simulink library "libEularAngleCalculator"  (R2016b)
settings: Solver=VariableStepAuto  StartTime=0.0  StopTime=10.0  RelTol=1e-3
libraries: simulink_extras x2
settings Model: Creator=vibek  LastModifiedBy=vibek

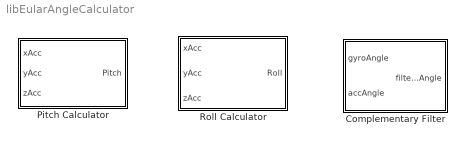
== system libEularAngleCalculator ==
  "Complementary Filter " : Subsystem
      mask DialogControl DescTextVar Prompt: Input Values of accelerometer and gyroscope angles to calculate filtered output angle
  Pitch Calculator : Subsystem  Description=takes 3 inputs from accelerometer and outputs pitch value
      settings: PermitHierarchicalResolution=None
      mask DialogControl DescTextVar Prompt: Input values of x, y, and z of Accelerometer data to calculate the value of Pitch
      mask Display: image('C:\Users\vibek\Pictures\93277-MG945-Servo-Motor-Metal-Gear-Tower-Pro-1-1200x630w.JPG');
  Roll Calculator : Subsystem  Description=takes 3 inputs from accelerometer and outputs pitch value
      mask DialogControl DescTextVar Prompt: Input values of x, y, and z of Accelerometer data to calculate the value of roll
      mask Display: image('C:\Users\vibek\Pictures\motor-tire.jpg');

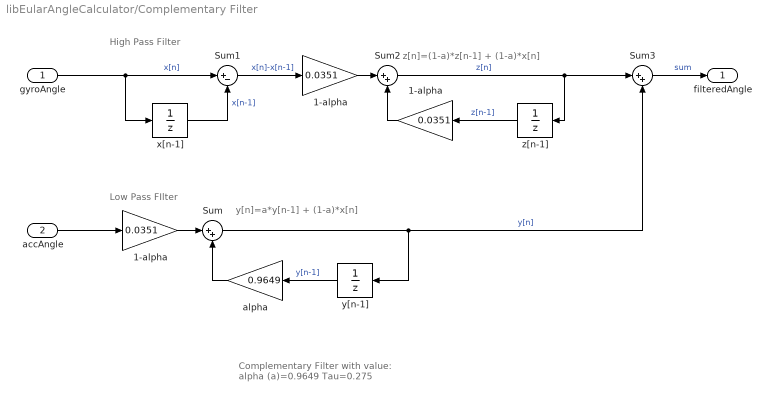
== system libEularAngleCalculator/Complementary Filter  ==
  note: Complementary Filter with value:
      | alpha (a)=0.9649
      | Tau=0.275
  note: y[n]=a*y[n-1] + (1-a)*x[n]
  note: Low Pass FIlter
  note: High Pass Filter
  note: z[n]=(1-a)*z[n-1] + (1-a)*x[n]
  gyroAngle : Inport
  accAngle : Inport  Port=2
  1-alpha : Gain  Gain=0.0351
  "1-alpha " : Gain  Gain=0.0351
  "1-alpha  " : Gain  Gain=0.0351
  Sum : Sum  Inputs=|++
  Sum1 : Sum  Inputs=|+-
  Sum2 : Sum  Inputs=|++
  Sum3 : Sum  Inputs=|++
  alpha : Gain  Gain=0.9649
  x[n-1] : UnitDelay  SampleTime=-1
  y[n-1] : UnitDelay  SampleTime=-1
  z[n-1] : UnitDelay  SampleTime=-1
  filteredAngle : Outport
  wires:
  accAngle/1 -> 1-alpha/1
  y[n-1]/1 -> alpha/1  "y[n-1]"
  1-alpha/1 -> Sum/1
  alpha/1 -> Sum/2
  Sum/1 -> Sum3/2, y[n-1]/1  "y[n]"
  gyroAngle/1 -> Sum1/1, x[n-1]/1  "x[n]"
  x[n-1]/1 -> Sum1/2  "x[n-1]"
  Sum1/1 -> "1-alpha "/1  "x[n]-x[n-1]"
  "1-alpha "/1 -> Sum2/1
  Sum2/1 -> Sum3/1, z[n-1]/1  "z[n]"
  z[n-1]/1 -> "1-alpha  "/1  "z[n-1]"
  "1-alpha  "/1 -> Sum2/2
  Sum3/1 -> filteredAngle/1  "sum"

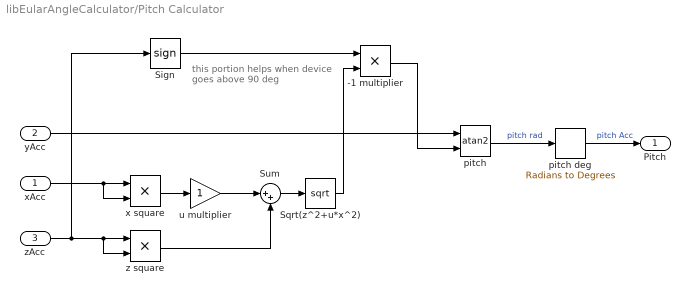
== system libEularAngleCalculator/Pitch Calculator ==
  note: this portion helps when device
      | goes above 90 deg
  xAcc : Inport
  yAcc : Inport  Port=2
  zAcc : Inport  Port=3
  -1 multiplier : Product
  Sign : Signum
  Sqrt(z^2+u*x^2) : Sqrt  SaturateOnIntegerOverflow=on
  Sum : Sum  Inputs=|++
  pitch : Trigonometry  Operator=atan2
  pitch deg : simulink_extras/Transformations/Radians to Degrees
  u multiplier : Gain
  x square : Product
  "z square " : Product
  Pitch : Outport
  wires:
  zAcc/1 -> "z square "/2, "z square "/1, Sign/1
  x square/1 -> u multiplier/1
  "z square "/1 -> Sum/2
  Sum/1 -> Sqrt(z^2+u*x^2)/1
  pitch/1 -> pitch deg/1  "pitch rad"
  pitch deg/1 -> Pitch/1  "pitch Acc"
  xAcc/1 -> x square/2, x square/1
  Sign/1 -> -1 multiplier/1
  Sqrt(z^2+u*x^2)/1 -> -1 multiplier/2
  -1 multiplier/1 -> pitch/2
  yAcc/1 -> pitch/1
  u multiplier/1 -> Sum/1

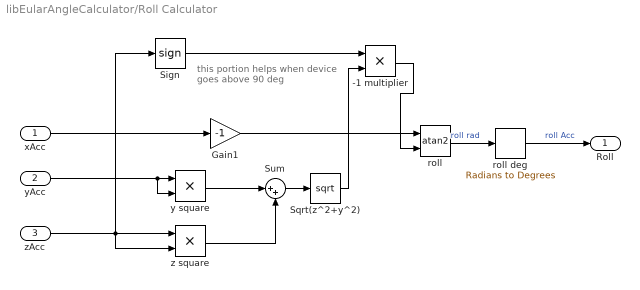
== system libEularAngleCalculator/Roll Calculator ==
  note: this portion helps when device
      | goes above 90 deg
  xAcc : Inport
  yAcc : Inport  Port=2
  zAcc : Inport  Port=3
  -1 multiplier : Product
  Gain1 : Gain  Gain=-1
  Sign : Signum
  Sqrt(z^2+y^2) : Sqrt  SaturateOnIntegerOverflow=on
  Sum : Sum  Inputs=|++
  roll : Trigonometry  Operator=atan2
  roll deg : simulink_extras/Transformations/Radians to Degrees
  y square : Product
  "z square " : Product
  Roll : Outport
  wires:
  yAcc/1 -> y square/2, y square/1
  zAcc/1 -> Sign/1, "z square "/1, "z square "/2
  "z square "/1 -> Sum/2
  Sqrt(z^2+y^2)/1 -> -1 multiplier/2
  Sign/1 -> -1 multiplier/1
  -1 multiplier/1 -> roll/2
  xAcc/1 -> Gain1/1
  y square/1 -> Sum/1
  Gain1/1 -> roll/1
  roll deg/1 -> Roll/1  "roll Acc"
  roll/1 -> roll deg/1  "roll rad"
  Sum/1 -> Sqrt(z^2+y^2)/1
